simulink model "top_level_faults"  (R2025b)
settings: Solver=FixedStepDiscrete  StartTime=0.0  StopTime=49.1  FixedStep=Ts  RelTol=1e-3
undefined symbols (not defined in the file): Ts
libraries: eeSequenceAnalyzer x6
settings Model: Creator=gdudgeon  LastModifiedBy=gdudgeon
settings DataIOCC: DSMLogging=off  InspectSignalLogs=on  SaveTime=off
settings ModelReferenceCC: UpdateModelReferenceTargets=AssumeUpToDate

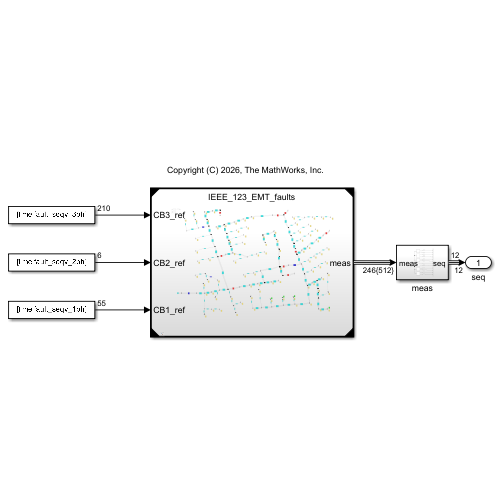
[thumbnail: Simulink's stored preview of the top-level diagram]
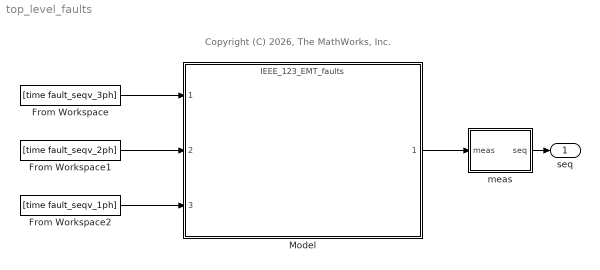
== system top_level_faults ==
  note: Copyright (C) 2026, The MathWorks, Inc.
  From Workspace : FromWorkspace  VariableName=[time fault_seqv_3ph]  SampleTime=Ts
  From Workspace1 : FromWorkspace  VariableName=[time fault_seqv_2ph]  SampleTime=Ts
  From Workspace2 : FromWorkspace  VariableName=[time fault_seqv_1ph]  SampleTime=Ts
  Model : ModelReference  ModelNameDialog=IEEE_123_EMT_faults.slx  ModelReferenceVersion=15.2
  meas : Subsystem
  seq : Outport
  wires:
  Model/1 -> meas/1(meas)
  meas/1(seq) -> seq/1
  From Workspace/1 -> Model/1
  From Workspace1/1 -> Model/2
  From Workspace2/1 -> Model/3

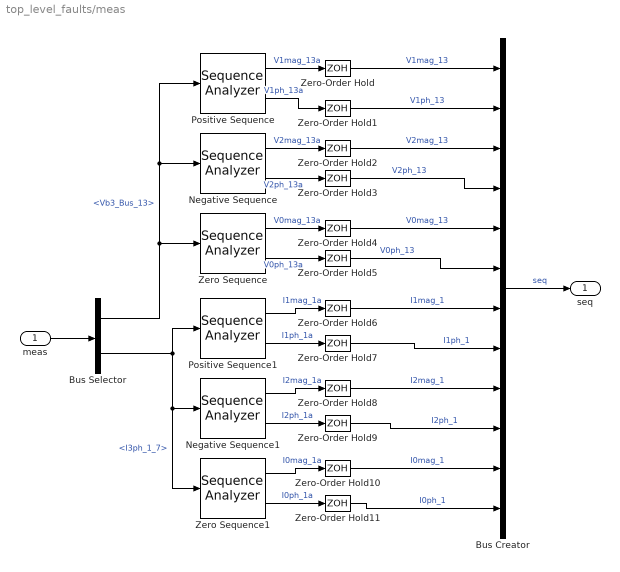
== system top_level_faults/meas ==
  meas : Inport
  Bus Creator : BusCreator  Inputs=12
  Bus Selector : BusSelector  OutputSignals=Vb3.Vb3_Bus_13,Il3.I3ph_1_7
  Negative Sequence : eeSequenceAnalyzer/Sequence Analyzer  VariantControl=Variant1  LabelModeActiveChoice=Discrete  F=60  K=1  Seq=Negative  Ts=Ts
      settings: LibrarySourceBlock=ee_sl_lib/Measurements/Sequence Analyzer
  Negative Sequence1 : eeSequenceAnalyzer/Sequence Analyzer  VariantControl=Variant1  LabelModeActiveChoice=Discrete  F=60  K=1  Seq=Negative  Ts=Ts
      settings: LibrarySourceBlock=ee_sl_lib/Measurements/Sequence Analyzer
  Positive Sequence : eeSequenceAnalyzer/Sequence Analyzer  VariantControl=Variant1  LabelModeActiveChoice=Discrete  F=60  K=1  Seq=Positive  Ts=Ts
      settings: LibrarySourceBlock=ee_sl_lib/Measurements/Sequence Analyzer
  Positive Sequence1 : eeSequenceAnalyzer/Sequence Analyzer  VariantControl=Variant1  LabelModeActiveChoice=Discrete  F=60  K=1  Seq=Positive  Ts=Ts
      settings: LibrarySourceBlock=ee_sl_lib/Measurements/Sequence Analyzer
  Zero Sequence : eeSequenceAnalyzer/Sequence Analyzer  VariantControl=Variant1  LabelModeActiveChoice=Discrete  F=60  K=1  Seq=Zero  Ts=Ts
      settings: LibrarySourceBlock=ee_sl_lib/Measurements/Sequence Analyzer
  Zero Sequence1 : eeSequenceAnalyzer/Sequence Analyzer  VariantControl=Variant1  LabelModeActiveChoice=Discrete  F=60  K=1  Seq=Zero  Ts=Ts
      settings: LibrarySourceBlock=ee_sl_lib/Measurements/Sequence Analyzer
  Zero-Order Hold{,1..11} (12 alike) : ZeroOrderHold  SampleTime=0.1
  seq : Outport
  wires:
  Bus Selector/1 -> Zero Sequence/1, Negative Sequence/1, Positive Sequence/1  "<Vb3_Bus_13>"
  Bus Selector/2 -> Zero Sequence1/1, Negative Sequence1/1, Positive Sequence1/1  "<I3ph_1_7>"
  Zero Sequence/2 -> Zero-Order Hold5/1  "V0ph_13a"
  Zero-Order Hold11/1 -> Bus Creator/12  "I0ph_1"
  Zero-Order Hold7/1 -> Bus Creator/8  "I1ph_1"
  Zero-Order Hold3/1 -> Bus Creator/4  "V2ph_13"
  Zero-Order Hold10/1 -> Bus Creator/11  "I0mag_1"
  Zero-Order Hold5/1 -> Bus Creator/6  "V0ph_13"
  Negative Sequence1/2 -> Zero-Order Hold9/1  "I2ph_1a"
  Zero Sequence/1 -> Zero-Order Hold4/1  "V0mag_13a"
  Zero-Order Hold1/1 -> Bus Creator/2  "V1ph_13"
  Zero-Order Hold6/1 -> Bus Creator/7  "I1mag_1"
  Negative Sequence/1 -> Zero-Order Hold2/1  "V2mag_13a"
  Zero-Order Hold4/1 -> Bus Creator/5  "V0mag_13"
  Positive Sequence/1 -> Zero-Order Hold/1  "V1mag_13a"
  Zero-Order Hold9/1 -> Bus Creator/10  "I2ph_1"
  Negative Sequence/2 -> Zero-Order Hold3/1  "V2ph_13a"
  Positive Sequence/2 -> Zero-Order Hold1/1  "V1ph_13a"
  Zero Sequence1/1 -> Zero-Order Hold10/1  "I0mag_1a"
  Negative Sequence1/1 -> Zero-Order Hold8/1  "I2mag_1a"
  Zero Sequence1/2 -> Zero-Order Hold11/1  "I0ph_1a"
  meas/1 -> Bus Selector/1
  Positive Sequence1/2 -> Zero-Order Hold7/1  "I1ph_1a"
  Positive Sequence1/1 -> Zero-Order Hold6/1  "I1mag_1a"
  Zero-Order Hold/1 -> Bus Creator/1  "V1mag_13"
  Zero-Order Hold2/1 -> Bus Creator/3  "V2mag_13"
  Zero-Order Hold8/1 -> Bus Creator/9  "I2mag_1"
  Bus Creator/1 -> seq/1  "seq"
